simulink model "UAV_Dynamics"  (R2023b)
settings: Solver=ode4  StartTime=0.0  StopTime=inf  RelTol=1e-3
model workspace (MAT data in the model file):
  Horizontal_position_accuracy = 0.01
  Horizontal_position_accuracy_fault : Simulink.Parameter (value not decoded)
  Velocity_accuracy = 0.01
  Velocity_accuracy_fault : Simulink.Parameter (value not decoded)
  Vertical_position_accuracy = 0.01
  Vertical_position_accuracy_fault : Simulink.Parameter (value not decoded)
  bias_acc = [0 0 0]
  bias_gyro = [0 0 0]
  mag_bias = [0 0 0]
undefined symbols (not defined in the file): contact, control, ddx, ddy, ddz, dragCoeffMov, dx, dy, dz, fractalcoef, g, m_to_mm, mass, p, pitch, q, r, ref_height, ref_lat, ref_lon, roll, rotorDir, rotorPositions, rotorThrustMax, rotorTimeConst, rotorTorqueMax, SampleTime, windVel, X, Y, yaw, Z
libraries: aerolibatmos2 x1, sensorgpslib x1, robotcorelib x1, mspsensorlib x1, shared6dof x1, simulink x1
(part 2 of 2)

== matlab function UAV_Dynamics/MATLAB Function3 ==
  data: inputFeatures input size=[1,23]; label output
function label = treeClassifier(inputFeatures)
% Funzione generata automaticamente da generateTreeCode
% inputFeatures: vettore di feature di input
% label: classe predetta

if inputFeatures(15) < -1.115931
    if inputFeatures(16) < 1.786899
        label = 0;
    else
        label = 4;
    end
else
    if inputFeatures(4) < 47.591815
        if inputFeatures(8) < 0.008461
            if inputFeatures(8) < -0.185740
                if inputFeatures(5) < 1.000336
                    if inputFeatures(23) < 0.002699
                        label = 0;
                    else
                        label = 2;
                    end
                else
                    if inputFeatures(8) < -0.206555
                        label = 2;
                    else
                        label = 0;
                    end
                end
            else
                if inputFeatures(7) < 0.026579
                    if inputFeatures(8) < -0.135154
                        if inputFeatures(4) < 46.978605
                            label = 0;
                        else
                            label = 3;
                        end
                    else
                        if inputFeatures(9) < 0.010693
                            label = 0;
                        else
                            if inputFeatures(14) < 1.150149
                                label = 0;
                            else
                                label = 1;
                            end
                        end
                    end
                else
                    if inputFeatures(5) < 1.000099
                        label = 2;
                    else
                        if inputFeatures(4) < 42.123060
                            label = 2;
                        else
                            if inputFeatures(22) < 37.058802
                                label = 0;
                            else
                                label = 1;
                            end
                        end
                    end
                end
            end
        else
            label = 1;
        end
    else
        if inputFeatures(1) < 1.075122
            label = 0;
        else
            label = 3;
        end
    end
end

end

== matlab function UAV_Dynamics/MATLAB Function1 ==
  data: inputMZ input; featuresVector output size=[1,23]; inputLAT input; inputLON input; inputAX input; inputGY input
function featuresVector = extractSelectedFeatures(inputMZ, inputLAT, inputLON, inputAX, inputGY)
    
    % Dimensioni del buffer
    bufferSize = 128;

    % Frequenza di campionamento (deve essere definita per i calcoli in frequenza)
    fs = 100; % Hz

    % Variabili persistenti per il buffering
    persistent bufferMZ bufferLAT bufferLON bufferAX bufferGY bufferIndex

    if isempty(bufferMZ)
        bufferMZ = zeros(bufferSize, 1);
        bufferLAT = zeros(bufferSize, 1);
        bufferLON = zeros(bufferSize, 1);
        bufferAX = zeros(bufferSize, 1);
        bufferGY = zeros(bufferSize, 1);
        bufferIndex = 1;
    end

    % Aggiorna il buffer
    bufferMZ(bufferIndex) = inputMZ;
    bufferLAT(bufferIndex) = inputLAT;
    bufferLON(bufferIndex) = inputLON;
    bufferAX(bufferIndex) = inputAX;
    bufferGY(bufferIndex) = inputGY;

    % Inizializza il vettore delle feature
    featuresVector = zeros(1, 23);

    if bufferIndex == bufferSize

        % Normalizza latitudine e longitudine
        normLAT = normalizeBuffer(bufferLAT);
        normLON = normalizeBuffer(bufferLON);

        % Calcola le feature per ogni segnale
        featuresVector(1:6) = calculateMZStatFeatures(bufferMZ);
        featuresVector(7) = calculateGYFeatures(bufferGY);       % Feature di GY (solo media)
        featuresVector(8:11) = calculateAXFeatures(bufferAX);          % Feature di AX (senza shape factor)
        featuresVector(12:15) = calculateStatFeatures(normLAT);       % Feature statistiche di LAT
        featuresVector(16:19) = calculateStatFeatures(normLON);      % Feature statistiche di LON
        featuresVector(20) = calculateBandPower(normLAT, fs); % Assegna un indice libero
        featuresVector(21) = calculateBandPower(normLON, fs);
        [featuresVector(22), featuresVector(23)] = calculateFreqFeatures(bufferGY, fs); % BandPower e PeakFreq di GY
        %[featuresVector(24), featuresVector(25)] = calculateFreqFeatures(bufferMZ, fs); % BandPower e PeakFreq di MZ
        
        bufferIndex = 1;
    else
        bufferIndex = bufferIndex + 1;
    end
    
end        

function normBuffer = normalizeBuffer(buffer)
    % Normalizza il buffer rispetto alla media e alla deviazione standard
    bufferMean = mean(buffer);
    bufferStd = std(buffer);
    if bufferStd == 0
        normBuffer = zeros(size(buffer)); % Restituisci un buffer normalizzato a 0
    else
        normBuffer = (buffer - bufferMean) / bufferStd;
    end
end


function bandPower = calculateBandPower(signal, fs)
    %#codegen

    % Parametri della funzione
    N = 128; % Numero di campioni
    fmin = 1;           % Banda di frequenza minima (Hz)
    fmax = 50;          % Banda di frequenza massima (Hz)

    % Calcolo dello spettro tramite FFT
    fftSignal = fft(signal, N);
    ps = abs(fftSignal).^2; % Spettro di potenza
    freqs = (0:N-1) * (fs / N); % Asse delle frequenze

    % Filtra solo la banda desiderata
    mask = (freqs >= fmin & freqs <= fmax);
    w_band = freqs(mask);
    ps_band = ps(mask);

    % BandPower
    bandPower = trapz(w_band, ps_band);

end

function [bandPower, peakFreq] = calculateFreqFeatures(signal, fs)
    %#codegen

    % Parametri della funzione
    N = 128; % Dimensione fissa
    fmin = 1; % Banda di frequenza minima (Hz)
    fmax = 50; % Banda di frequenza massima (Hz)

    % Calcolo dello spettro tramite FFT
    fftSignal = fft(signal, N);
    ps = abs(fftSignal).^2; % Spettro di potenza
    freqs = (0:N-1) * (fs / N); % Asse delle frequenze

    % Filtra solo la banda desiderata
    mask = (freqs >= fmin & freqs <= fmax);
    w_band = freqs(mask);
    ps_band = ps(mask);

    % BandPower
    bandPower = trapz(w_band, ps_band);

    % PeakFreq
    [~, idx] = max(ps_band);
    peakFreq = w_band(idx);
end


function features = calculateAXFeatures(signal)
    % Feature di AX: mean, max, rms, std
    features = [mean(signal), max(signal), rms(signal), std(signal)];
end

function features = calculateStatFeatures(signal)
    % Calcola feature statistiche: clearance factor, crest factor,
    % impulse factor, kurtosis, peak value, shape factor, skewness
    features = [crestFactor(signal), ...
                max(signal), ...
                shapeFactor(signal), ...
                skewnessCalc(signal)];
end

function features = calculateGYFeatures(signal)
    % Feature di GY: solo mean
    features = mean(signal);
end

% Funzioni per calcolare i vari indici statistici
function cl = clearanceFactor(signal)
    cl = max(abs(signal)) / mean(sqrt(abs(signal)));
end

function cf = crestFactor(signal)
    cf = max(abs(signal)) / rms(signal);
end

function imp = impulseFactor(signal)
    imp = max(abs(signal)) / mean(abs(signal));
end

function sf = shapeFactor(signal)
    sf = rms(signal) / mean(abs(signal));
end

function sk = skewnessCalc(signal)
    sk = mean((signal - mean(signal)).^3) / (std(signal)^3);
end

function features = calculateMZStatFeatures(signal)
    features = [clearanceFactor(signal), crestFactor(signal), impulseFactor(signal), max(signal), shapeFactor(signal), std(signal)];
end

== matlab function UAV_Dynamics/Buffer1/MATLAB Function2 ==
  data: buffer input; orderedBuffer output; k input
function orderedBuffer = readCircularBuffer(buffer, k)
    % Funzione per leggere un buffer circolare in ordine
    % buffer: il buffer circolare corrente (array)
    % k: indice dell'inizio del buffer circolare
 
    bufferSize = length(buffer); % Ottieni la dimensione del buffer
    orderedBuffer = zeros(1, bufferSize); % Prealloca il buffer ordinato
 
    % Riordina il buffer partendo dall'indice k
    for i = 1:bufferSize
        orderedBuffer(i) = buffer(k);
        k = mod(k, bufferSize) + 1; % Aggiorna l'indice circolare
    end
end

== matlab function UAV_Dynamics/Buffer2/MATLAB Function ==
  data: buffer input; buffer output; newValue input; bufferSize input; k input; k output
function [buffer, k] = writeCircularBuffer(buffer, newValue, bufferSize, k)

    % Funzione per implementare un buffer circolare con indice
    % buffer: il buffer corrente (array)
    % newValue: il nuovo valore da aggiungere
    % bufferSize: la dimensione massima del buffer
    % k: indice dell'inizio del buffer circolar
 
    % Inserisci il nuovo valore nella posizione corretta
    buffer(k) = newValue;
 
    % Aggiorna l'indice k per il prossimo elemento
    k = mod(k, bufferSize) + 1;
end

== matlab function UAV_Dynamics/Buffer2/MATLAB Function2 ==
  data: buffer input; orderedBuffer output; k input
function orderedBuffer = readCircularBuffer(buffer, k)
    % Funzione per leggere un buffer circolare in ordine
    % buffer: il buffer circolare corrente (array)
    % k: indice dell'inizio del buffer circolare
 
    bufferSize = length(buffer); % Ottieni la dimensione del buffer
    orderedBuffer = zeros(1, bufferSize); % Prealloca il buffer ordinato
 
    % Riordina il buffer partendo dall'indice k
    for i = 1:bufferSize
        orderedBuffer(i) = buffer(k);
        k = mod(k, bufferSize) + 1; % Aggiorna l'indice circolare
    end
end

== matlab function UAV_Dynamics/Buffer3/MATLAB Function ==
  data: buffer input; buffer output; newValue input; bufferSize input; k input; k output
function [buffer, k] = writeCircularBuffer(buffer, newValue, bufferSize, k)

    % Funzione per implementare un buffer circolare con indice
    % buffer: il buffer corrente (array)
    % newValue: il nuovo valore da aggiungere
    % bufferSize: la dimensione massima del buffer
    % k: indice dell'inizio del buffer circolar
 
    % Inserisci il nuovo valore nella posizione corretta
    buffer(k) = newValue;
 
    % Aggiorna l'indice k per il prossimo elemento
    k = mod(k, bufferSize) + 1;
end

== matlab function UAV_Dynamics/Buffer3/MATLAB Function2 ==
  data: buffer input; orderedBuffer output; k input
function orderedBuffer = readCircularBuffer(buffer, k)
    % Funzione per leggere un buffer circolare in ordine
    % buffer: il buffer circolare corrente (array)
    % k: indice dell'inizio del buffer circolare
 
    bufferSize = length(buffer); % Ottieni la dimensione del buffer
    orderedBuffer = zeros(1, bufferSize); % Prealloca il buffer ordinato
 
    % Riordina il buffer partendo dall'indice k
    for i = 1:bufferSize
        orderedBuffer(i) = buffer(k);
        k = mod(k, bufferSize) + 1; % Aggiorna l'indice circolare
    end
end

== matlab function UAV_Dynamics/Buffer4/MATLAB Function ==
  data: buffer input; buffer output; newValue input; bufferSize input; k input; k output
function [buffer, k] = writeCircularBuffer(buffer, newValue, bufferSize, k)

    % Funzione per implementare un buffer circolare con indice
    % buffer: il buffer corrente (array)
    % newValue: il nuovo valore da aggiungere
    % bufferSize: la dimensione massima del buffer
    % k: indice dell'inizio del buffer circolar
 
    % Inserisci il nuovo valore nella posizione corretta
    buffer(k) = newValue;
 
    % Aggiorna l'indice k per il prossimo elemento
    k = mod(k, bufferSize) + 1;
end

== matlab function UAV_Dynamics/Buffer4/MATLAB Function2 ==
  data: buffer input; orderedBuffer output; k input
function orderedBuffer = readCircularBuffer(buffer, k)
    % Funzione per leggere un buffer circolare in ordine
    % buffer: il buffer circolare corrente (array)
    % k: indice dell'inizio del buffer circolare
 
    bufferSize = length(buffer); % Ottieni la dimensione del buffer
    orderedBuffer = zeros(1, bufferSize); % Prealloca il buffer ordinato
 
    % Riordina il buffer partendo dall'indice k
    for i = 1:bufferSize
        orderedBuffer(i) = buffer(k);
        k = mod(k, bufferSize) + 1; % Aggiorna l'indice circolare
    end
end

== matlab function UAV_Dynamics/Buffer5/MATLAB Function ==
  data: buffer input; buffer output; newValue input; bufferSize input; k input; k output
function [buffer, k] = writeCircularBuffer(buffer, newValue, bufferSize, k)

    % Funzione per implementare un buffer circolare con indice
    % buffer: il buffer corrente (array)
    % newValue: il nuovo valore da aggiungere
    % bufferSize: la dimensione massima del buffer
    % k: indice dell'inizio del buffer circolar
 
    % Inserisci il nuovo valore nella posizione corretta
    buffer(k) = newValue;
 
    % Aggiorna l'indice k per il prossimo elemento
    k = mod(k, bufferSize) + 1;
end

== matlab function UAV_Dynamics/Buffer5/MATLAB Function2 ==
  data: buffer input; orderedBuffer output; k input
function orderedBuffer = readCircularBuffer(buffer, k)
    % Funzione per leggere un buffer circolare in ordine
    % buffer: il buffer circolare corrente (array)
    % k: indice dell'inizio del buffer circolare
 
    bufferSize = length(buffer); % Ottieni la dimensione del buffer
    orderedBuffer = zeros(1, bufferSize); % Prealloca il buffer ordinato
 
    % Riordina il buffer partendo dall'indice k
    for i = 1:bufferSize
        orderedBuffer(i) = buffer(k);
        k = mod(k, bufferSize) + 1; % Aggiorna l'indice circolare
    end
end

== matlab function UAV_Dynamics/MATLAB Function2 ==
  data: bufferMZ input; featuresVector output size=[1,23]; bufferLAT input; bufferLON input; bufferAX input; bufferGY input
 function featuresVector = extractSelectedFeatures(bufferMZ, bufferLAT, bufferLON, bufferAX, bufferGY)


    % Frequenza di campionamento (deve essere definita per i calcoli in frequenza)
    fs = 100; % Hz

    % Inizializza il vettore delle feature
    featuresVector = zeros(1, 23);
    
        % Normalizza latitudine e longitudine
        normLAT = normalizeBuffer(bufferLAT);
        normLON = normalizeBuffer(bufferLON);


        % Calcola le feature per ogni segnale
        featuresVector(1:6) = calculateMZStatFeatures(bufferMZ);
        featuresVector(7) = calculateGYFeatures(bufferGY);       % Feature di GY (solo media)
        featuresVector(8:11) = calculateAXFeatures(bufferAX);          % Feature di AX (senza shape factor)
        featuresVector(12:15) = calculateStatFeatures(normLAT);       % Feature statistiche di LAT
        featuresVector(16:19) = calculateStatFeatures(normLON);      % Feature statistiche di LON
        featuresVector(20) = calculateBandPower(normLAT, fs); % Assegna un indice libero
        featuresVector(21) = calculateBandPower(normLON, fs);
        [featuresVector(22), featuresVector(23)] = calculateFreqFeatures(bufferGY, fs); % BandPower e PeakFreq di GY
    
end        

function normBuffer = normalizeBuffer(buffer)
    % Normalizza il buffer rispetto alla media e alla deviazione standard
    bufferMean = mean(buffer);
    bufferStd = std(buffer);
    if bufferStd == 0
        normBuffer = zeros(size(buffer)); % Restituisci un buffer normalizzato a 0
    else
        normBuffer = (buffer - bufferMean) / bufferStd;
    end
end


function bandPower = calculateBandPower(signal, fs)
    %#codegen

    % Parametri della funzione
    N = 128; % Numero di campioni
    fmin = 1;           % Banda di frequenza minima (Hz)
    fmax = 50;          % Banda di frequenza massima (Hz)

    % Calcolo dello spettro tramite FFT
    fftSignal = fft(signal, N);
    ps = abs(fftSignal).^2; % Spettro di potenza
    freqs = (0:N-1) * (fs / N); % Asse delle frequenze

    % Filtra solo la banda desiderata
    mask = (freqs >= fmin & freqs <= fmax);
    w_band = freqs(mask);
    ps_band = ps(mask);

    % BandPower
    bandPower = trapz(w_band, ps_band);

end

function [bandPower, peakFreq] = calculateFreqFeatures(signal, fs)
    %#codegen

    % Parametri della funzione
    N = 128; % Dimensione fissa
    fmin = 1; % Banda di frequenza minima (Hz)
    fmax = 50; % Banda di frequenza massima (Hz)

    % Calcolo dello spettro tramite FFT
    fftSignal = fft(signal, N);
    ps = abs(fftSignal).^2; % Spettro di potenza
    freqs = (0:N-1) * (fs / N); % Asse delle frequenze

    % Filtra solo la banda desiderata
    mask = (freqs >= fmin & freqs <= fmax);
    w_band = freqs(mask);
    ps_band = ps(mask);

    % BandPower
    bandPower = trapz(w_band, ps_band);

    % PeakFreq
    [~, idx] = max(ps_band);
    peakFreq = w_band(idx);
end


function features = calculateAXFeatures(signal)
    % Feature di AX: mean, max, rms, std
    features = [mean(signal), max(signal), rms(signal), std(signal)];
end

function features = calculateStatFeatures(signal)
    % Calcola feature statistiche: clearance factor, crest factor,
    % impulse factor, kurtosis, peak value, shape factor, skewness
    features = [crestFactor(signal), ...
                max(signal), ...
                shapeFactor(signal), ...
                skewnessCalc(signal)];
end

function features = calculateGYFeatures(signal)
    % Feature di GY: solo mean
    features = mean(signal);
end

% Funzioni per calcolare i vari indici statistici
function cl = clearanceFactor(signal)
    cl = max(abs(signal)) / mean(sqrt(abs(signal)));
end

function cf = crestFactor(signal)
    cf = max(abs(signal)) / rms(signal);
end

function imp = impulseFactor(signal)
    imp = max(abs(signal)) / mean(abs(signal));
end

function sf = shapeFactor(signal)
    sf = rms(signal) / mean(abs(signal));
end

function sk = skewnessCalc(signal)
    sk = mean((signal - mean(signal)).^3) / (std(signal)^3);
end

function features = calculateMZStatFeatures(signal)
    features = [clearanceFactor(signal), crestFactor(signal), impulseFactor(signal), max(signal), shapeFactor(signal), std(signal)];
end

== matlab function UAV_Dynamics/MATLAB Function ==
  data: currentLabel input; filteredLabel output
function filteredLabel = filterUsingBuffer(currentLabel)
    %#codegen

    % Dimensione del buffer
    bufferSize = 500;

    % Variabili persistenti per memorizzare il buffer e l'indice corrente
    persistent labelBuffer bufferIndex

    % Inizializza il buffer alla prima esecuzione
    if isempty(labelBuffer)
        labelBuffer = zeros(bufferSize, 1); % Buffer di stringhe inizializzato a vuoto
        bufferIndex = 1; % Indice per la scrittura nel buffer
    end

    % Inserisce l'etichetta corrente nel buffer in modo circolare
    labelBuffer(bufferIndex) = currentLabel;
    bufferIndex = mod(bufferIndex, bufferSize) + 1; % Incrementa l'indice (circolare)

    % Trova la modalità (l'etichetta più frequente nel buffer)
    uniqueLabels = unique(labelBuffer); % Etichette uniche nel buffer
    labelCounts = zeros(size(uniqueLabels)); % Contatori per ciascuna etichetta

    for i = 1:length(uniqueLabels)
        labelCounts(i) = sum(labelBuffer == uniqueLabels(i)); % Conta le occorrenze
    end

    % Trova l'etichetta con il massimo conteggio
    [~, maxIdx] = max(labelCounts);
    filteredLabel = uniqueLabels(maxIdx); % Etichetta più frequente
end

== matlab function UAV_Dynamics/actuators_faults/MATLAB Function ==
  data: input input size=4; tf input; currentTime input; output output; num_motore input; loss_effectiveness input; perc input; lock_in_place input; prec_output input; float input; hardover input
function output   = FaultMotor(input , tf, currentTime, num_motore , loss_effectiveness, ...
    perc, lock_in_place, prec_output, float, hardover)


    output = input;
    if (currentTime >= tf)

        if lock_in_place
            if num_motore == 0
                output = input ;
            else
                output(num_motore) = prec_output(num_motore);
            end 
        end
        
        if float
            if num_motore == 0
                output = input;
            else
                output(num_motore) = 0;
            end  
        end
       
        
        if hardover
            if num_motore == 0
                output = input ;
            else
                output(num_motore) = 1;
            end 
        end
        
        if loss_effectiveness
            if num_motore == 0
                output = input ;
            else
                output(num_motore) = output(num_motore) - (perc / 100)* output(num_motore);
            end 
        end
    end
end

== matlab function UAV_Dynamics/acc_faults/MATLAB Function ==
  settings: updateMethod=DISCRETE
  data: tf input; drift input; landa input; freezing input; accuracy input; d_accuracy input; bias input; bias_values input; prec_output input; currentTime input; input input; output output
function output = fault_acc(tf, drift, landa, freezing, accuracy, d_accuracy, bias, bias_values, ...
    prec_output, currentTime, input)

    % output preallocation
    output = input;

    % check the fault time
    if currentTime >= tf
        % calculete the time from the start of the fault
        time_since_fault = currentTime - tf;

        % ---- Linear Drift  ----
        if any(drift)
            if drift(1) % Drift  X
                output(1) = output(1) + landa * time_since_fault;
            end
            if drift(2) % Drift  Y
                output(2) = output(2) + landa * time_since_fault;
            end
            if drift(3) % Drift  Z
                output(3) = output(3) + landa * time_since_fault;
            end
        end

        % ---- Accuracy ----
        if any(accuracy)
            if accuracy(1) % Accuracy  X
                output(1) = output(1) + ((rand - 0.5) * 2) * d_accuracy;
            end
            if accuracy(2) % Accuracy  Y
                output(2) = output(2) + ((rand - 0.5) * 2) * d_accuracy;
            end
            if accuracy(3) % Accuracy  Z
                output(3) = output(3) + ((rand - 0.5) * 2) * d_accuracy;
            end
        end

        % ---- Freezing ----
        if any(freezing)
            if freezing(1) % Freezing X
                output(1) = prec_output(1);
            end
            if freezing(2) % Freezing  Y
                output(2) = prec_output(2);
            end
            if freezing(3) % Freezing  Z
                output(3) = prec_output(3);
            end
        end

        % ---- Bias ----
        if any(bias)
            if bias(1) % Bias X
                output(1) = output(1) + bias_values(1);
            end
            if bias(2) % Bias Y
                output(2) = output(2) + bias_values(2);
            end
            if bias(3) % Bias Z
                output(3) = output(3) + bias_values(3);
            end
        end
    end
end

== matlab function UAV_Dynamics/gyro_faults/MATLAB Function ==
  settings: updateMethod=DISCRETE
  data: tf input; drift input; landa input; freezing input; accuracy input; d_accuracy input; bias input; bias_values input; prec_output input; currentTime input; input input; output output
function output = fault_gyro(tf, drift, landa, freezing, accuracy, d_accuracy, bias, bias_values, ...
    prec_output, currentTime, input)

    % Preallocazione dell'output
    output = input;

    % Controlla se il tempo corrente è maggiore o uguale al tempo di guasto
    if currentTime >= tf
        % Calcola il tempo relativo dall'inizio del guasto
        time_since_fault = currentTime - tf;

        % ---- Drift Lineare ----
        if any(drift)
            if drift(1) % Drift lungo X
                output(1) = output(1) + landa * time_since_fault;
            end
            if drift(2) % Drift lungo Y
                output(2) = output(2) + landa * time_since_fault;
            end
            if drift(3) % Drift lungo Z
                output(3) = output(3) + landa * time_since_fault;
            end
        end

        % ---- Accuratezza ----
        if any(accuracy)
            if accuracy(1) % Accuratezza lungo X
                output(1) = output(1) + ((rand - 0.5) * 2) * d_accuracy;
            end
            if accuracy(2) % Accuratezza lungo Y
                output(2) = output(2) + ((rand - 0.5) * 2) * d_accuracy;
            end
            if accuracy(3) % Accuratezza lungo Z
                output(3) = output(3) + ((rand - 0.5) * 2) * d_accuracy;
            end
        end

        % ---- Freezing ----
        if any(freezing)
            if freezing(1) % Freezing lungo X
                output(1) = prec_output(1);
            end
            if freezing(2) % Freezing lungo Y
                output(2) = prec_output(2);
            end
            if freezing(3) % Freezing lungo Z
                output(3) = prec_output(3);
            end
        end

        % ---- Bias ----
        if any(bias)
            if bias(1) % Bias lungo X
                output(1) = output(1) + bias_values(1);
            end
            if bias(2) % Bias lungo Y
                output(2) = output(2) + bias_values(2);
            end
            if bias(3) % Bias lungo Z
                output(3) = output(3) + bias_values(3);
            end
        end
    end
end

== matlab function UAV_Dynamics/mag_faults/MATLAB Function ==
  settings: updateMethod=DISCRETE
  data: tf input; drift input; landa input; freezing input; accuracy input; d_accuracy input; bias input; bias_values input; prec_output input; currentTime input; input input; output output
function output = fault_mag(tf, drift, landa, freezing, accuracy, d_accuracy, bias, bias_values, ...
    prec_output, currentTime, input)

    % Preallocazione dell'output
    output = input;

    % Controlla se il tempo corrente è maggiore o uguale al tempo di guasto
    if currentTime >= tf
        % Calcola il tempo relativo dall'inizio del guasto
        time_since_fault = currentTime - tf;

        % ---- Drift Lineare ----
        if any(drift)
            if drift(1) % Drift lungo X
                output(1) = output(1) + landa * time_since_fault;
            end
            if drift(2) % Drift lungo Y
                output(2) = output(2) + landa * time_since_fault;
            end
            if drift(3) % Drift lungo Z
                output(3) = output(3) + landa * time_since_fault;
            end
        end

        % ---- Accuratezza ----
        if any(accuracy)
            if accuracy(1) % Accuratezza lungo X
                output(1) = output(1) + ((rand - 0.5) * 2) * d_accuracy;
            end
            if accuracy(2) % Accuratezza lungo Y
                output(2) = output(2) + ((rand - 0.5) * 2) * d_accuracy;
            end
            if accuracy(3) % Accuratezza lungo Z
                output(3) = output(3) + ((rand - 0.5) * 2) * d_accuracy;
            end
        end

        % ---- Freezing ----
        if any(freezing)
            if freezing(1) % Freezing lungo X
                output(1) = prec_output(1);
            end
            if freezing(2) % Freezing lungo Y
                output(2) = prec_output(2);
            end
            if freezing(3) % Freezing lungo Z
                output(3) = prec_output(3);
            end
        end

        % ---- Bias ----
        if any(bias)
            if bias(1) % Bias lungo X
                output(1) = output(1) + bias_values(1);
            end
            if bias(2) % Bias lungo Y
                output(2) = output(2) + bias_values(2);
            end
            if bias(3) % Bias lungo Z
                output(3) = output(3) + bias_values(3);
            end
        end
    end
end

== matlab function UAV_Dynamics/Quadcopter Model/Force and Moment Calculation/Rotor Model/MATLAB Function ==
  data: thrustEachRotor input; tauEachRotor input; rotorPositions input; netF output; netM output; rotorDir input
function [netF, netM] = getForceMoment(thrustEachRotor, tauEachRotor, rotorPositions, rotorDir)
%#codegen
Fx = 0;
Fy = 0;
Fz = -sum(thrustEachRotor);

netF = [Fx; Fy; Fz];

netM = [0; 0; 0]; %initialize
    for i = 1:4
        rotPos = rotorPositions(:, i);
        Fi = [0, 0, -thrustEachRotor(i)]';
        netM = netM +  cross(rotPos, Fi);%contribution from thrusts of each propeller
        netM(3) = netM(3) - rotorDir(i)*tauEachRotor(i); %contribution from counter torque acting on propeller
    end

end
